simulink model "sim_mpc"  (R2025a)
settings: Solver=FixedStepAuto  StartTime=0.0  StopTime=sim_time  FixedStep=0.001  RelTol=1e-3
undefined symbols (not defined in the file): accl, accl_param_limit, accl_param_n, alpha, base_alpha, base_time, coulomb_friction, counter, decel, delay_n, dist, ego_accl, ego_alpha, ego_dist, ego_state, ego_v, ego_w, end_v, end_w, ff_duty_low_th, ff_duty_low_v_th, gear_ratio, k1, k2, k_theta, k_x, k_y, ke, km, limit_time_count, lm, mass, param_alpha, pow_n, resist, sla, sla_param, slip, slip_gain, state, test_mode, tgt_angle, tgt_dist, tire, tread, trj_length, v, v_max, viscous_friction, vx, w, w_max
settings Model: Creator=nao12  LastModifiedBy=naoto
settings SolverCC: AlgebraicLoopSolver=TrustRegion
settings DataIOCC: SaveOutput=off  SignalLogging=off  DSMLogging=off  SaveTime=off  ReturnWorkspaceOutputs=off
settings OptimizationCC: DefaultParameterBehavior=Inlined  StrengthReduction=on  PassReuseOutputArgsAs=Individual arguments  ZeroExternalMemoryAtStartup=off  ZeroInternalMemoryAtStartup=off  OptimizeBlockOrder=speed  OptimizationPriority=Speed  OptimizationCustomize=off  MultiThreadedLoops=on  AutoScheduleForLoops=on  EfficientTunableParamExpr=on
settings DebuggingCC: ParameterTunabilityLossMsg=error  UnconnectedInputMsg=warning  UnconnectedOutputMsg=warning  UnconnectedLineMsg=warning  ArithmeticOperatorsInVariantConditions=warning
settings HardwareCC: ProdBitPerPointer=32.0  ProdBitPerSizeT=32.0  ProdBitPerPtrDiffT=32.0  ProdLargestAtomicFloat=None  ProdWordSize=32.0  ProdHWDeviceType=Renesas->RX
settings ModelReferenceCC: UpdateModelReferenceTargets=IfOutOfDate  EnableRefExpFcnMdlSchedulingChecks=on
settings SFSimCC: SimCustomHeaderCode="#include \"bus.h\""  SimUserIncludeDirs=../include/  MATLABDynamicMemAlloc=off  CustomCodeUndefinedFunction=UseInterfaceOnly
settings RTWCC: SystemTargetFile=ert.tlc  GenCodeOnly=on  TemplateMakefile=ert_default_tmf  GenerateReport=on  RTWUseSimCustomCode=on  CustomHeaderCode="#include \"bus.h\""  CustomInclude=../include/  IncludeHyperlinkInReport=on  LaunchReport=on  TargetLang=C++  GenerateTraceInfo=on  GenerateTraceReport=on  GenerateTraceReportSl=on  GenerateTraceReportSf=on  GenerateTraceReportEml=on  GenerateCodeMetricsReport=on  GPUComputeCapability=3.5  DLArmComputeVersion=19.05  Description=Embedded Coder
settings CodeAppCC: ForceParamTrailComments=on  IgnoreCustomStorageClasses=off  OperatorAnnotations=on  SimulinkDataObjDesc=on  SFDataObjDesc=on  InsertBlockDesc=on
settings ERTTargetCC: ExtModeTransport=0.0  ExtModeStaticAlloc=off  ExtModeMexFile=ext_comm  ExtModeIntrfLevel=Level1  RootIOFormat=Structure reference  ERTCustomFileTemplate=example_file_process.tlc  EnableUserReplacementTypes=on  DynamicArrayContainerType=coder::array  TargetLangStandard=C++17 (ISO)  GenerateSampleERTMain=on  SupportAbsoluteTime=off  CodeInterfacePackaging=C++ class  SubcomponentCodeInterfacePackaging=C++ class  SupportComplex=off
settings SimscapeCC: SimscapeLogDecimation=1  SimscapeLogDataHistory=5000

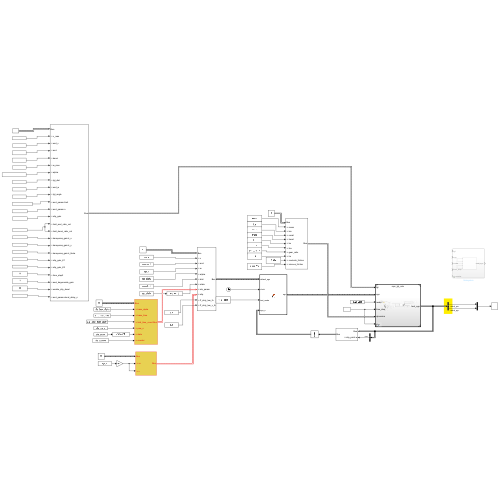
[thumbnail: Simulink's stored preview of the top-level diagram]
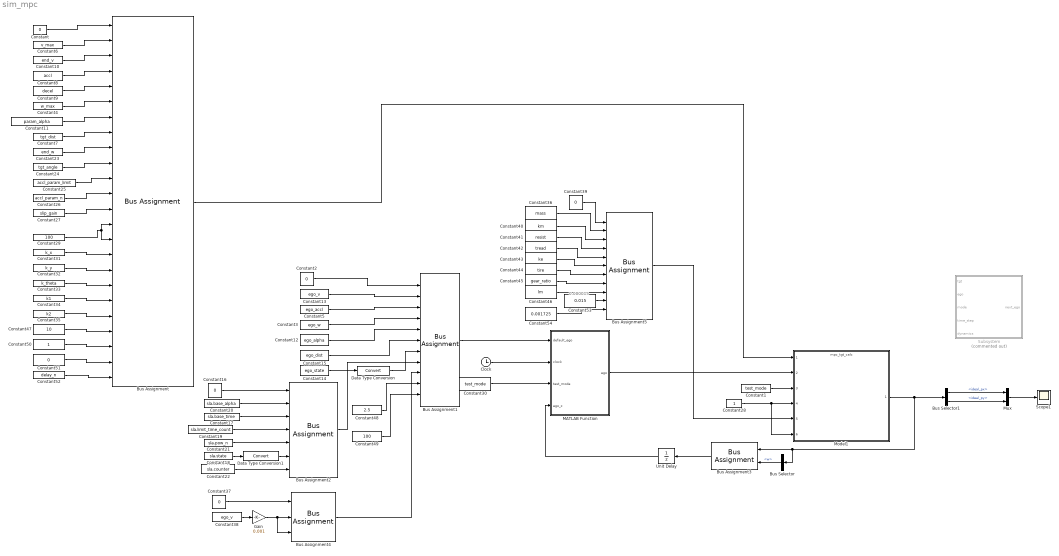
== system sim_mpc ==
  note: 0.000015
  Bus Assignment : BusAssignment  AssignedSignals=v_max,end_v,accl,decel,w_max,alpha,tgt_dist,end_w,tgt_angle,accl_param.limit,accl_param.n,slip_gain,limit_accl_ratio_cnt,limit_decel_ratio_cnt,kanayama_gain.k_x,kanayama_gain.k_y,kanayama_gain.k_theta,slip_gain_K1,slip_gain_K2,time_step2,axel_degenerate_gain,enable_slip_decel,accl_param.decel_delay_n
  Bus Assignment1 : BusAssignment  AssignedSignals=v,accl,w,alpha,dist,state,sla_param,slip,ff_duty_low_th,ff_duty_low_v_th
  Bus Assignment2 : BusAssignment  AssignedSignals=base_alpha,base_time,limit_time_count,pow_n,state,counter
  Bus Assignment3 : BusAssignment  AssignedSignals=slip_point.w
  Bus Assignment4 : BusAssignment  AssignedSignals=vx,v
  Bus Assignment5 : BusAssignment  AssignedSignals=mass,km,resist,tread,ke,tire,gear_ratio,lm,coulomb_friction,viscous_friction
  Bus Selector : BusSelector  OutputSignals=w
  Bus Selector1 : BusSelector  OutputSignals=ideal_px,ideal_py
  Clock : Clock
  Constant : Constant  Value=0  OutDataTypeStr=Bus: t_tgt
  Constant1 : Constant  Value=test_mode  OutDataTypeStr=int32
  Constant10 : Constant  Value=end_v  OutDataTypeStr=single
  Constant11 : Constant  Value=param_alpha  OutDataTypeStr=single
  Constant12 : Constant  Value=ego_alpha  OutDataTypeStr=single
  Constant13 : Constant  Value=ego_v  OutDataTypeStr=single
  Constant14 : Constant  Value=ego_state
  Constant15 : Constant  Value=ego_dist  OutDataTypeStr=single
  Constant16 : Constant  Value=0  OutDataTypeStr=Bus: t_slalom
  Constant17 : Constant  Value=sla.base_time  OutDataTypeStr=single
  Constant18 : Constant  Value=sla.state  OutDataTypeStr=int8
  Constant19 : Constant  Value=sla.limit_time_count  OutDataTypeStr=single
  Constant2 : Constant  Value=0  OutDataTypeStr=Bus: t_ego
  Constant20 : Constant  Value=sla.base_alpha  OutDataTypeStr=single
  Constant21 : Constant  Value=sla.pow_n  OutDataTypeStr=single
  Constant22 : Constant  Value=sla.counter  OutDataTypeStr=int32
  Constant23 : Constant  Value=end_w  OutDataTypeStr=single
  Constant24 : Constant  Value=tgt_angle  OutDataTypeStr=single
  Constant25 : Constant  Value=accl_param_limit  OutDataTypeStr=single
  Constant26 : Constant  Value=accl_param_n  OutDataTypeStr=single
  Constant27 : Constant  Value=slip_gain  OutDataTypeStr=single
  Constant28 : Constant  OutDataTypeStr=int32
  Constant29 : Constant  Value=100  OutDataTypeStr=single
  Constant3 : Constant  Value=ego_w  OutDataTypeStr=single
  Constant30 : Constant  Value=test_mode  OutDataTypeStr=int32
  Constant31 : Constant  Value=k_x  OutDataTypeStr=single
  Constant32 : Constant  Value=k_y  OutDataTypeStr=single
  Constant33 : Constant  Value=k_theta  OutDataTypeStr=single
  Constant34 : Constant  Value=k1  OutDataTypeStr=single
  Constant35 : Constant  Value=k2  OutDataTypeStr=single
  Constant36 : Constant  Value=mass  OutDataTypeStr=single
  Constant37 : Constant  Value=0  OutDataTypeStr=Bus: t_slip
  Constant38 : Constant  Value=ego_v  OutDataTypeStr=single
  Constant39 : Constant  Value=0  OutDataTypeStr=Bus: t_dynamics
  Constant4 : Constant  Value=w_max  OutDataTypeStr=single
  Constant40 : Constant  Value=km  OutDataTypeStr=single
  Constant41 : Constant  Value=resist  OutDataTypeStr=single
  Constant42 : Constant  Value=tread  OutDataTypeStr=single
  Constant43 : Constant  Value=ke  OutDataTypeStr=single
  Constant44 : Constant  Value=tire  OutDataTypeStr=single
  Constant45 : Constant  Value=gear_ratio  OutDataTypeStr=single
  Constant46 : Constant  Value=lm  OutDataTypeStr=single
  Constant47 : Constant  Value=10  OutDataTypeStr=int32
  Constant48 : Constant  Value=2.5  OutDataTypeStr=single
  Constant49 : Constant  Value=100  OutDataTypeStr=single
  Constant5 : Constant  Value=ego_accl  OutDataTypeStr=single
  Constant50 : Constant  OutDataTypeStr=single
  Constant51 : Constant  Value=0  OutDataTypeStr=int8
  Constant52 : Constant  Value=delay_n  OutDataTypeStr=single
  Constant53 : Constant  Value=0.015  OutDataTypeStr=single
  Constant54 : Constant  Value=0.001725  OutDataTypeStr=single
  Constant6 : Constant  Value=v_max  OutDataTypeStr=single
  Constant7 : Constant  Value=tgt_dist  OutDataTypeStr=single
  Constant8 : Constant  Value=accl  OutDataTypeStr=single
  Constant9 : Constant  Value=decel  OutDataTypeStr=single
  Data Type Conversion : DataTypeConversion  SaturateOnIntegerOverflow=off  RndMeth=Floor
  Data Type Conversion1 : DataTypeConversion  SaturateOnIntegerOverflow=off  RndMeth=Floor
  Gain : Gain  Gain=0.001
  MATLAB Function : MATLAB Function  TreatAsAtomicUnit=on
  Model1 : ModelReference  ModelNameDialog=mpc_tgt_calc.slx  SimulationMode=Normal  ModelReferenceVersion=11.8
  Mux : Mux  Inputs=2
  Scope1 : Scope
      settings: ActiveDisplayYMinimum=-25.692067806076071  ActiveDisplayYMaximum=45.488327384124943
  Subsystem : Subsystem  Commented=on
  Unit Delay : UnitDelay  SampleTime=-1  HasFrameUpgradeWarning=on
  wires:
  Constant/1 -> Bus Assignment/1
  Bus Assignment/1 -> Model1/1
  Constant1/1 -> Model1/3
  Constant2/1 -> Bus Assignment1/1
  Bus Assignment1/1 -> MATLAB Function/1(default_ego)
  Constant6/1 -> Bus Assignment/2
  Constant8/1 -> Bus Assignment/4
  Constant9/1 -> Bus Assignment/5
  Constant4/1 -> Bus Assignment/6
  Constant11/1 -> Bus Assignment/7
  Constant7/1 -> Bus Assignment/8
  Constant10/1 -> Bus Assignment/3
  Constant13/1 -> Bus Assignment1/2
  Constant3/1 -> Bus Assignment1/4
  Constant5/1 -> Bus Assignment1/3
  Constant12/1 -> Bus Assignment1/5
  Constant15/1 -> Bus Assignment1/6
  Constant14/1 -> Data Type Conversion/1
  Constant16/1 -> Bus Assignment2/1
  Bus Assignment2/1 -> Bus Assignment1/8
  Constant20/1 -> Bus Assignment2/2
  Constant17/1 -> Bus Assignment2/3
  Constant19/1 -> Bus Assignment2/4
  Constant18/1 -> Data Type Conversion1/1
  Constant21/1 -> Bus Assignment2/5
  Constant22/1 -> Bus Assignment2/7
  Constant23/1 -> Bus Assignment/9
  Constant24/1 -> Bus Assignment/10
  Clock/1 -> MATLAB Function/2(clock)
  Unit Delay/1 -> MATLAB Function/4(ego_z)
  Constant25/1 -> Bus Assignment/11
  Constant26/1 -> Bus Assignment/12
  Constant27/1 -> Bus Assignment/13
  Constant28/1 -> Model1/4, Model1/6
  Bus Assignment3/1 -> Unit Delay/1
  Bus Selector/1 -> Bus Assignment3/2  "<w>"
  Constant29/1 -> Bus Assignment/14, Bus Assignment/15
  Constant30/1 -> MATLAB Function/3(test_mode)
  Constant31/1 -> Bus Assignment/16
  Constant32/1 -> Bus Assignment/17
  Constant33/1 -> Bus Assignment/18
  Data Type Conversion/1 -> Bus Assignment1/7
  Data Type Conversion1/1 -> Bus Assignment2/6
  Constant34/1 -> Bus Assignment/19
  Constant35/1 -> Bus Assignment/20
  Constant36/1 -> Bus Assignment5/2
  MATLAB Function/1(ego) -> Model1/2
  Bus Assignment4/1 -> Bus Assignment1/9
  Constant37/1 -> Bus Assignment4/1
  Constant38/1 -> Gain/1
  Gain/1 -> Bus Assignment4/3, Bus Assignment4/2
  Constant39/1 -> Bus Assignment5/1
  Constant40/1 -> Bus Assignment5/3
  Constant41/1 -> Bus Assignment5/4
  Constant42/1 -> Bus Assignment5/5
  Constant43/1 -> Bus Assignment5/6
  Constant44/1 -> Bus Assignment5/7
  Constant45/1 -> Bus Assignment5/8
  Bus Assignment5/1 -> Model1/5
  Constant46/1 -> Bus Assignment5/9
  Constant47/1 -> Bus Assignment/21
  Constant48/1 -> Bus Assignment1/10
  Constant49/1 -> Bus Assignment1/11
  Constant50/1 -> Bus Assignment/22
  Constant51/1 -> Bus Assignment/23
  Constant52/1 -> Bus Assignment/24
  Constant53/1 -> Bus Assignment5/10
  Constant54/1 -> Bus Assignment5/11
  Model1/1 -> Bus Selector/1, Bus Assignment3/1, Bus Selector1/1
  Mux/1 -> Scope1/1
  Bus Selector1/1 -> Mux/1  "<ideal_px>"
  Bus Selector1/2 -> Mux/2  "<ideal_py>"

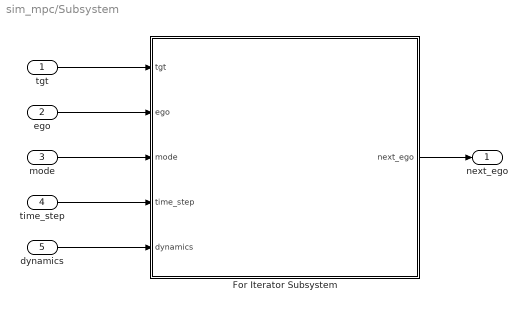
== system sim_mpc/Subsystem ==
  tgt : Inport
  ego : Inport  Port=2
  mode : Inport  Port=3
  time_step : Inport  Port=4
  dynamics : Inport  Port=5
  For Iterator Subsystem : Subsystem  TreatAsAtomicUnit=on
  next_ego : Outport
  wires:
  tgt/1 -> For Iterator Subsystem/1(tgt)
  ego/1 -> For Iterator Subsystem/2(ego)
  mode/1 -> For Iterator Subsystem/3(mode)
  time_step/1 -> For Iterator Subsystem/4(time_step)
  dynamics/1 -> For Iterator Subsystem/5(dynamics)
  For Iterator Subsystem/1(next_ego) -> next_ego/1

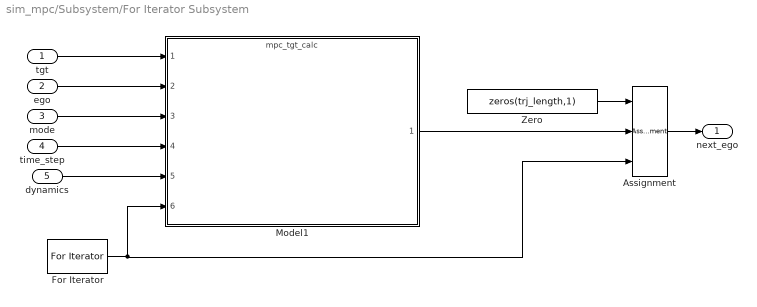
== system sim_mpc/Subsystem/For Iterator Subsystem ==
  tgt : Inport
  ego : Inport  Port=2
  mode : Inport  Port=3
  time_step : Inport  Port=4
  dynamics : Inport  Port=5
  Assignment : Assignment  DiagnosticForDimensions=Warning  IndexOptions=Index vector (port)  Indices=1  OutputSizes=1
  For Iterator : ForIterator  IterationLimit=trj_length
  Model1 : ModelReference  ModelNameDialog=mpc_tgt_calc.slx  SimulationMode=Normal  ModelReferenceVersion=11.8
  Zero : Constant  Value=zeros(trj_length,1)  OutDataTypeStr=Bus: t_ego
  next_ego : Outport  OutDataTypeStr=Bus: t_ego
  wires:
  ego/1 -> Model1/2
  mode/1 -> Model1/3
  Assignment/1 -> next_ego/1
  Model1/1 -> Assignment/2
  dynamics/1 -> Model1/5
  Zero/1 -> Assignment/1
  For Iterator/1 -> Model1/6, Assignment/3
  tgt/1 -> Model1/1
  time_step/1 -> Model1/4

== matlab function sim_mpc/MATLAB Function ==
  data: default_ego input; ego output Bus: t_ego; clock input; test_mode input; ego_z input; sim_time parameter
function ego  = fcn( default_ego, clock, test_mode, ego_z, sim_time)
   ego = debug( default_ego, clock, ego_z, test_mode, sim_time);
end
